simulink model "unitdelay_sampletime"  (R2023b)
settings: Solver=FixedStepAuto  StartTime=0.0  StopTime=10.0  RelTol=1e-3
settings Model: Creator=hp  LastModifiedBy=hp

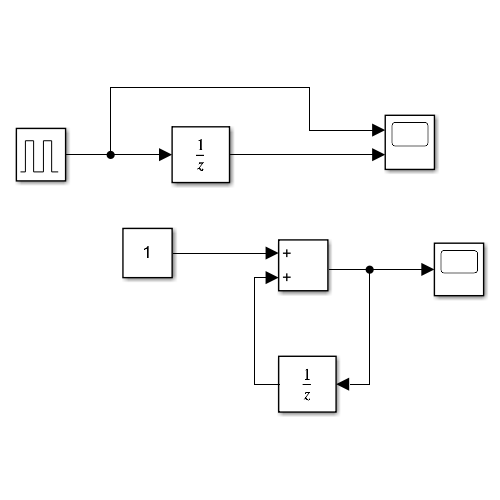
[thumbnail: Simulink's stored preview of the top-level diagram]
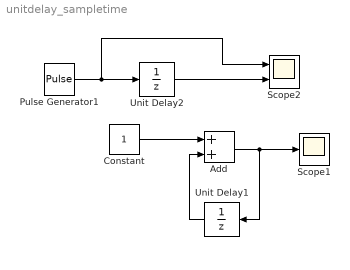
== system unitdelay_sampletime ==
  Add : Sum
  Constant : Constant
  Pulse Generator1 : DiscretePulseGenerator  PulseType=Time based  Period=1  PulseWidth=50
  Scope1 : Scope
  Scope2 : Scope  NumInputPorts=2
  Unit Delay1 : UnitDelay  SampleTime=-1  HasFrameUpgradeWarning=on
  Unit Delay2 : UnitDelay  SampleTime=-1  HasFrameUpgradeWarning=on
  wires:
  Unit Delay2/1 -> Scope2/2
  Pulse Generator1/1 -> Unit Delay2/1, Scope2/1
  Add/1 -> Unit Delay1/1, Scope1/1
  Unit Delay1/1 -> Add/2
  Constant/1 -> Add/1
